simulink model "buck_converter_CPM_closed_loop"  (R2016a)
settings: Solver=ode23tb  StartTime=0.0  StopTime=0.5  MaxStep=1/fs  RelTol=1/fs
values from neighbouring files (symbols this model uses):
  C = 680e-6    (= 0.00068)    [buck_converter_CPM_parameters.m]
  Dmax = 0.9    [buck_converter_CPM_parameters.m]
  Dmin = 0    [buck_converter_CPM_parameters.m]
  fs = 200e3    (= 200000)    [buck_converter_CPM_parameters.m]
  Gcv0 = Gcvwc/abs(1+wz/(i*wc))    [buck_converter_CPM_parameters.m]
  H = 0.6    [buck_converter_CPM_parameters.m]
  L = 45e-6    (= 4.5e-05)    [buck_converter_CPM_parameters.m]
  Resr = 0.8e-3    (= 0.0008)    [buck_converter_CPM_parameters.m]
  RL = 15e-3    (= 0.015)    [buck_converter_CPM_parameters.m]
  Rload = Vo/Io    (= 0.288)    [buck_converter_CPM_parameters.m]
  Rs = 0.1    [buck_converter_CPM_parameters.m]
  Va = Rs*ma*(1/fs)    (= 0.133333333333)    [buck_converter_CPM_parameters.m]
  Vcc = 5    [buck_converter_CPM_parameters.m]
  Vcmax = Vcc    (= 5)    [buck_converter_CPM_parameters.m]
  Vg = 48    [buck_converter_CPM_parameters.m]
  Vo = 12    [buck_converter_CPM_parameters.m]
  Voffset = 0    [buck_converter_CPM_parameters.m]
  wz = 2*pi*fz    (= 62831.8530718)    [buck_converter_CPM_parameters.m]
libraries: simulink x3, simulink_extras x1
settings Model: Creator=Gorkem  LastModifiedBy=Gorkem
settings GRTTargetCC: GeneratePreprocessorConditionals=Use local settings

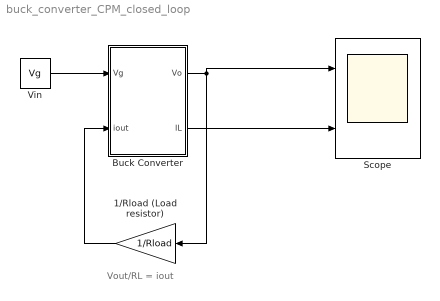
== system buck_converter_CPM_closed_loop ==
  note: Vout/RL = iout
  1/Rload (Load resistor) : Gain  Gain=1/Rload
  Buck Converter : Subsystem
  Scope : Scope  NumInputPorts=2
  Vin : Constant  Value=Vg
  wires:
  Buck Converter/1(Vo) -> Scope/1, 1/Rload (Load resistor)/1
  1/Rload (Load resistor)/1 -> Buck Converter/2(iout)
  Vin/1 -> Buck Converter/1(Vg)
  Buck Converter/2(IL) -> Scope/2

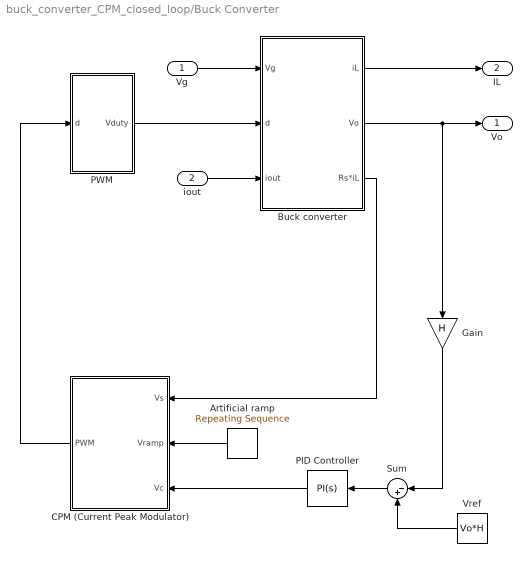
== system buck_converter_CPM_closed_loop/Buck Converter ==
  Vg : Inport
  iout : Inport  Port=2
  Artificial ramp : simulink/Sources/Repeating Sequence  rep_seq_t=[0 0.999/fs 1/fs]  rep_seq_y=[0 Va 0]
  Buck converter : Subsystem
  CPM (Current Peak Modulator) : Subsystem
  Gain : Gain  Gain=H
  PID Controller : simulink/Continuous/PID Controller  Controller=PI  TimeDomain=Continuous-time  SampleTime=-1  IntegratorMethod=Forward Euler  FilterMethod=Forward Euler  Form=Parallel  UseFilter=on  ControllerParametersSource=internal  P=Gcv0  I=Gcv0*wz  D=0  N=100  InitialConditionSource=internal  InitialConditionForIntegrator=0  InitialConditionForFilter=0  ExternalReset=none  LimitOutput=off  UpperSaturationLimit=inf  LowerSaturationLimit=-inf  LinearizeAsGain=on  AntiWindupMode=none  Kb=1  TrackingMode=off  Kt=1  PParamMin=[]  PParamMax=[]  IParamMin=[]  IParamMax=[]  DParamMin=[]  DParamMax=[]  NParamMin=[]  NParamMax=[]  KbParamMin=[]  KbParamMax=[]  KtParamMin=[]  KtParamMax=[]  POutMin=[]  POutMax=[]  IOutMin=[]  IOutMax=[]  DOutMin=[]  DOutMax=[]  NOutMin=[]  NOutMax=[]  KbOutMin=[]  KbOutMax=[]  KtOutMin=[]  KtOutMax=[]  IntegratorOutMin=[]  IntegratorOutMax=[]  FilterOutMin=[]  FilterOutMax=[]  SumOutMin=[]  SumOutMax=[]  SumI1OutMin=[]  SumI1OutMax=[]  SumI2OutMin=[]  SumI2OutMax=[]  SumI3OutMin=[]  SumI3OutMax=[]  SumDOutMin=[]  SumDOutMax=[]  SaturationOutMin=[]  SaturationOutMax=[]  IntegratorContinuousStateAttributes=''  IntegratorStateMustResolveToSignalObject=off  IntegratorRTWStateStorageClass=Auto  FilterContinuousStateAttributes=''  FilterStateMustResolveToSignalObject=off  FilterRTWStateStorageClass=Auto  DifferentiatorICPrevScaledInput=0  DifferentiatorOutMin=[]  DifferentiatorOutMax=[]
  PWM : Subsystem
  Sum : Sum  Inputs=|-+
  Vref : Constant  Value=Vo*H
  Vo : Outport
  IL : Outport  Port=2
  wires:
  Artificial ramp/1 -> CPM (Current Peak Modulator)/2(Vramp)
  Buck converter/3(Rs*iL) -> CPM (Current Peak Modulator)/1(Vs)
  PID Controller/1 -> CPM (Current Peak Modulator)/3(Vc)
  iout/1 -> Buck converter/3(iout)
  Vref/1 -> Sum/2
  PWM/1(Vduty) -> Buck converter/2(d)
  Gain/1 -> Sum/1
  Vg/1 -> Buck converter/1(Vg)
  CPM (Current Peak Modulator)/1(PWM) -> PWM/1(d)
  Buck converter/1(iL) -> IL/1
  Sum/1 -> PID Controller/1
  Buck converter/2(Vo) -> Vo/1, Gain/1

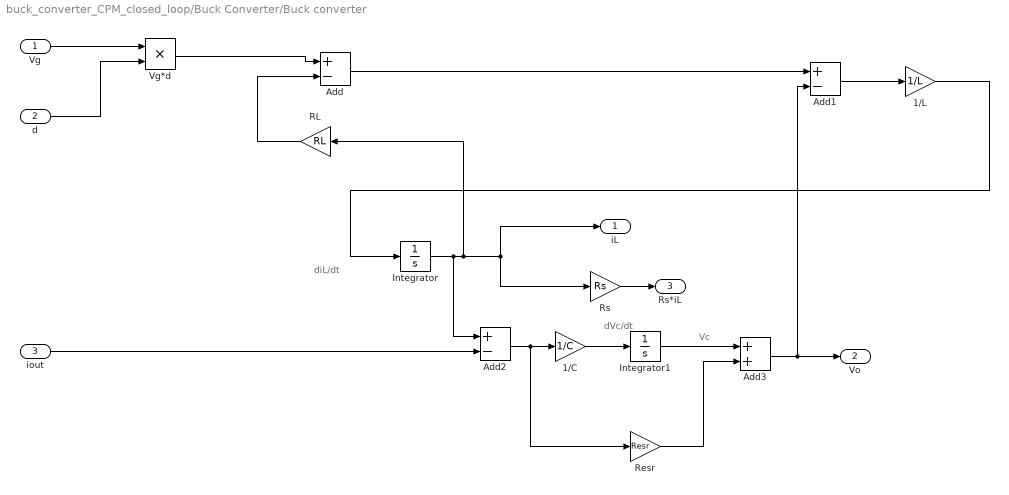
== system buck_converter_CPM_closed_loop/Buck Converter/Buck converter ==
  note: Vc
  note: dVc/dt
  note: diL/dt
  Vg : Inport
  d : Inport  Port=2
  iout : Inport  Port=3
  1/C : Gain  Gain=1/C
  1/L : Gain  Gain=1/L
  Add : Sum  Inputs=+-
  Add1 : Sum  Inputs=+-
  Add2 : Sum  Inputs=+-
  Add3 : Sum
  Integrator : Integrator
  Integrator1 : Integrator
  RL : Gain  Gain=RL
  Resr : Gain  Gain=Resr
  Rs : Gain  Gain=Rs
  Vg*d : Product
  iL : Outport
  Vo : Outport  Port=2
  Rs*iL : Outport  Port=3
  wires:
  1/L/1 -> Integrator/1
  Integrator/1 -> Add2/1, Rs/1, iL/1, RL/1
  Vg/1 -> Vg*d/1
  1/C/1 -> Integrator1/1
  Add2/1 -> Resr/1, 1/C/1
  Vg*d/1 -> Add/1
  Add1/1 -> 1/L/1
  Add3/1 -> Vo/1, Add1/2
  d/1 -> Vg*d/2
  Integrator1/1 -> Add3/1
  Resr/1 -> Add3/2
  RL/1 -> Add/2
  iout/1 -> Add2/2
  Add/1 -> Add1/1
  Rs/1 -> Rs*iL/1

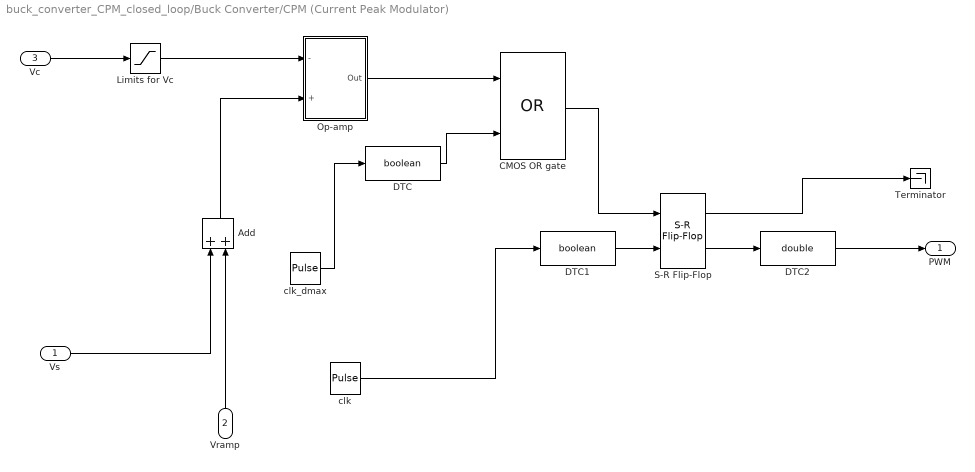
== system buck_converter_CPM_closed_loop/Buck Converter/CPM (Current Peak Modulator) ==
  Vs : Inport
  Vramp : Inport  Port=2
  Vc : Inport  Port=3
  Add : Sum
  CMOS OR gate : Logic  Operator=OR  AllPortsSameDT=off  OutDataTypeStr=boolean
  DTC : DataTypeConversion  OutDataTypeStr=boolean  SaturateOnIntegerOverflow=on  LockScale=on
  DTC1 : DataTypeConversion  OutDataTypeStr=boolean  SaturateOnIntegerOverflow=on  LockScale=on
  DTC2 : DataTypeConversion  OutDataTypeStr=double  SaturateOnIntegerOverflow=on  LockScale=on
  Limits for Vc : Saturate  UpperLimit=Vcmax+Voffset  LowerLimit=0  ZeroCross=off
  Op-amp : Subsystem
  S-R Flip-Flop : simulink_extras/Flip Flops/S-R Flip-Flop  initial_condition=0
  Terminator : Terminator
  clk : DiscretePulseGenerator  PulseType=Time based  Amplitude=5  Period=1/fs  PulseWidth=(Dmin+1e-10)*100
  clk_dmax : DiscretePulseGenerator  PulseType=Time based  Amplitude=5  Period=1/fs  PulseWidth=(1-Dmax)*100  PhaseDelay=Dmax/fs
  PWM : Outport
  wires:
  Vs/1 -> Add/1
  Add/1 -> Op-amp/2(+)
  Limits for Vc/1 -> Op-amp/1(-)
  Vramp/1 -> Add/2
  Vc/1 -> Limits for Vc/1
  S-R Flip-Flop/2 -> DTC2/1
  CMOS OR gate/1 -> S-R Flip-Flop/1
  clk_dmax/1 -> DTC/1
  DTC/1 -> CMOS OR gate/2
  DTC1/1 -> S-R Flip-Flop/2
  clk/1 -> DTC1/1
  S-R Flip-Flop/1 -> Terminator/1
  Op-amp/1(Out) -> CMOS OR gate/1
  DTC2/1 -> PWM/1

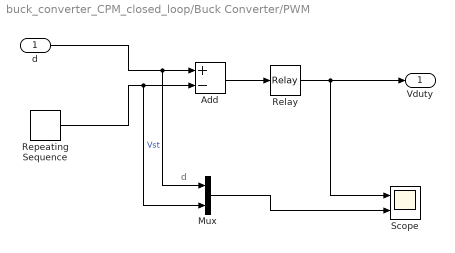
== system buck_converter_CPM_closed_loop/Buck Converter/PWM ==
  note: d
  d : Inport
  Add : Sum  Inputs=+-
  Mux : Mux  Inputs=2
  Relay : Relay  ZeroCross=off
  Repeating Sequence : simulink/Sources/Repeating Sequence  rep_seq_t=[0 0.001e-5 1/fs]  rep_seq_y=[1 0 1]
  Scope : Scope  NumInputPorts=2
  Vduty : Outport
  wires:
  Relay/1 -> Vduty/1, Scope/1
  Repeating Sequence/1 -> Mux/2, Add/2  "Vst"
  Add/1 -> Relay/1
  Mux/1 -> Scope/2
  d/1 -> Mux/1, Add/1

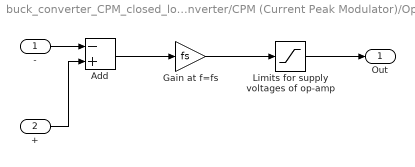
== system buck_converter_CPM_closed_loop/Buck Converter/CPM (Current Peak Modulator)/Op-amp ==
  - : Inport
  + : Inport  Port=2
  Add : Sum  Inputs=-+
  Gain at f=fs : Gain  Gain=fs
  "Limits for supply voltages of op-amp " : Saturate  UpperLimit=Vcc  LowerLimit=0
  Out : Outport
  wires:
  Add/1 -> Gain at f=fs/1
  Gain at f=fs/1 -> "Limits for supply voltages of op-amp "/1
  "Limits for supply voltages of op-amp "/1 -> Out/1
  -/1 -> Add/1
  +/1 -> Add/2
